simulink model "MatchedfilterImproved"  (R2023b)
settings: Solver=VariableStepAuto  StartTime=0.0  StopTime=4000/fs  RelTol=1e-3
PreLoadFcn:
  | fs = 16e6;
  | 
  | % Test tone
  | f = 0.2*16e6;
  | 
  | % Parameters
  | N = 2048;
  | n = 0:N-1;
  | 
  | % Windows
  | Hamming = 0.54 - 0.46 * cos(2*pi*n/N);
  | Norm_Ham = sum(Hamming);
  | Hanning = 0.5 * (1 + cos(2*pi*n/N));
  | Norm_Han = sum(Hanning);
values from neighbouring files (symbols this model uses):
  template = fliplr(conj(template))    [MF_startup.m]
libraries: hdlBasic x46, hdlDSPIP x3, hdlsllib x2, vmcUtilities x1
settings Model: Creator=qsb20164  LastModifiedBy=jojok
settings DebuggingCC: UnconnectedInputMsg=warning  UnconnectedOutputMsg=warning  UnconnectedLineMsg=warning
settings ModelReferenceCC: EnableRefExpFcnMdlSchedulingChecks=on
settings RTWCC: DLArmComputeVersion=19.05

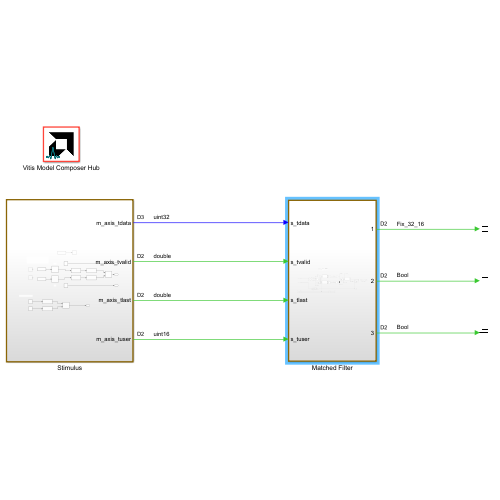
[thumbnail: Simulink's stored preview of the top-level diagram]
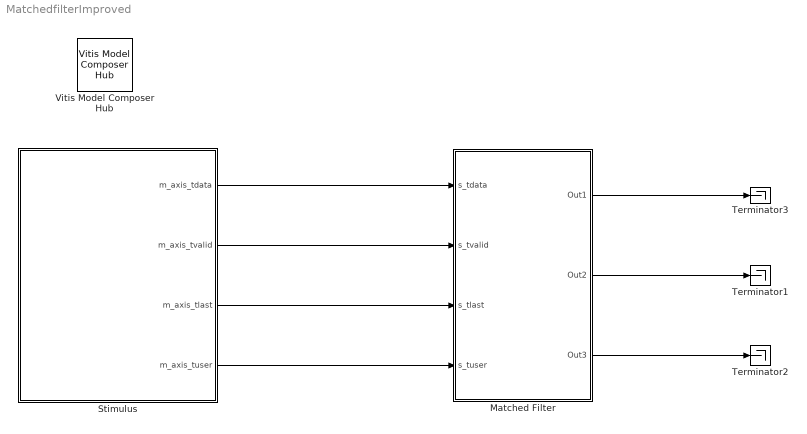
== system MatchedfilterImproved ==
  Matched Filter : Subsystem
  Stimulus : Subsystem
  Terminator1 : Terminator
  Terminator2 : Terminator
  Terminator3 : Terminator
  Vitis Model Composer Hub : vmcUtilities/Vitis Model Composer Hub  Tag=genX  CodeGeneration=off  SubsystemName=Matched Filter  DUTSubsystemName=Matched Filter  CompilationType=HDLCompilation  ExportTypeV2=IP Catalog  TargetDirectory=./ImprovedMFnetlist\ip\Matched_Filter\src  exportDesign=on  analyzeDesign=off  validateDesignOnHw=off  ExportType=HDL  IpVendor=xilinx.com  IpLibrary=hls  IpVersion=1.0  IpHWLanguage=Verilog  AieCompilerOptions={}  AieSimulatorOptions={}  CreateTestbench=off  TestbenchStackSize=10  RunRtlSim=off  RunCSim=off  RunAieSim=off  AieSimTimeout=50000  RunAieSimProfiling=off  LaunchVitisAnalyzer=off  PlotOutput=off  RunX86Sim=off  X86SimTimeout=10  GenHwImage=off  GenLibadfXo=on  GenHwValidationCode=off  PlatformType=Not Specified  HwSystemType=Baremetal  HwValidationTarget=hw  ProjDevice=xczu28dr-ffvg1517-2-e  ProjDevicePart=xczu28dr-ffvg1517-2-e  SamplePeriod=-1  ClockFrequency=200  DataPathParallelism=1  xilinxfamily=zynquplusRFSOC  part=xczu28dr  speed=-2-e  package=ffvg1517  directory=./netlist\ip\Matched_Filter\src  testbench=off  incr_netlist=off  synthesis_tool=Vivado  clock_wrapper=Clock Enables  dbl_ovrd=According to Block Masks  dcm_input_clock_period=10  sysclk_period=4  simulink_period=1/(2*fs)  eval_field=0  IPInfoJsonString="{\"HDLSubsystem\":{\"SubsystemName\":\"Matched_Filter\",\"IPName\":\"Matched_Filter\",\"IPLibrary\":\"VMC\",\"IPVendor\":\"User Company\",\"IPVersion\":\"1.0\",\"TargetDirectory\":\"./ImprovedMFnetlist\",\"SubsystemDir\":\"./ImprovedMFnetlist\\\\ip\\\\Matched_Filter\"},\"SubsystemTag\":\"HDLNode\"}"  LogFileName=''  NThreads=4
  wires:
  Stimulus/1(m_axis_tdata) -> Matched Filter/1(s_tdata)
  Stimulus/2(m_axis_tvalid) -> Matched Filter/2(s_tvalid)
  Stimulus/3(m_axis_tlast) -> Matched Filter/3(s_tlast)
  Matched Filter/1(Out1) -> Terminator3/1
  Matched Filter/2(Out2) -> Terminator1/1
  Matched Filter/3(Out3) -> Terminator2/1
  Stimulus/4(m_axis_tuser) -> Matched Filter/4(s_tuser)

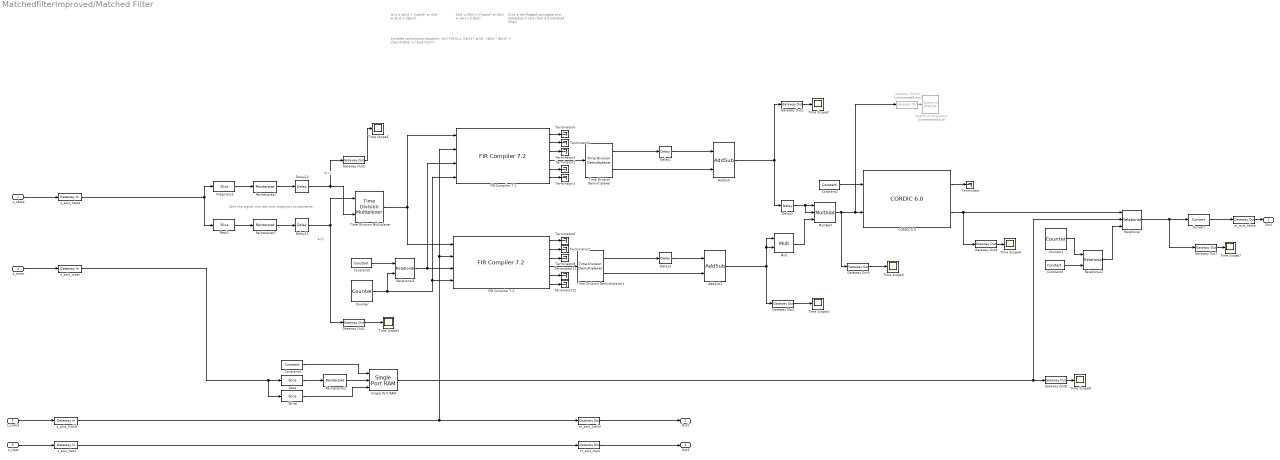
== system MatchedfilterImproved/Matched Filter ==
  note: a[n]
  note: b[n]
  note: h[n] is the flipped conjugate
      | of a template in x[n]
      | (this is a matched filter)
  note: h[n] = hl[n] + j(hq[n])
      | or
      | h[n] = c[n] + j(d[n])
  note: x[n] = xl[n] + j(xq[n])
      | or
      | x[n] = a[n] + j(b[n])
  note: Complex convolution equation:
      |
      | x[n] * h[n] = ((a[n] * c[n]) - (b[n] * d[n])) + j((a[n]*d[n]) + (b[n]*c[n]))
  note: Split the signal into real and imaginary components
  s_tdata : Inport
  s_tvalid : Inport  Port=2
  s_tlast : Inport  Port=3
  s_tuser : Inport  Port=4
  AddSub : hdlBasic/AddSub  mode=Subtraction  use_carryin=off  use_carryout=off  en=off  latency=1  precision=Full  arith_type=Unsigned  n_bits=16  bin_pt=14  quantization=Truncate  overflow=Wrap  use_behavioral_HDL=off  hw_selection=Fabric  pipelined=off  XmcBlockStatus=1  maskContainerNames=tabcontainer1  block_type=addsub  block_config=sysgen:Addsub_config
  AddSub1 : hdlBasic/AddSub  mode=Addition  use_carryin=off  use_carryout=off  en=off  latency=1  precision=Full  arith_type=Unsigned  n_bits=16  bin_pt=14  quantization=Truncate  overflow=Wrap  use_behavioral_HDL=off  hw_selection=Fabric  pipelined=off  XmcBlockStatus=1  maskContainerNames=tabcontainer1  block_type=addsub  block_config=sysgen:Addsub_config
  CORDIC 6.0 : hdlDSPIP/CORDIC 6.0   functional_selection=Square_Root  architectural_configuration=Parallel  pipelining_mode=Maximum  data_format=UnsignedInteger  phase_format=Radians  input_width=46  output_width=24  round_mode=Truncate  iterations=0  precision=0  compensation_scaling=No_Scale_Compensation  coarse_rotation=off  aclken=off  aresetn=off  out_tready=off  cartesian_has_tuser=off  cartesian_has_tlast=off  cartesian_tuser_width=1  phase_has_tuser=off  phase_has_tlast=off  phase_tuser_width=1  out_tlast_behv=Null  flow_control=NonBlocking  optimize_goal=Resources  trim_axipin_name=on  simulation_type=hybrid_sim  simulation_model=sysgen:cordic_v6_0  data_path_portlist={'s_axis_cartesian_tdata_imag', 's_axis_cartesian_tdata_real', 's_axis_phase_tdata_phase', 'm_axis_dout_tdata_imag', 'm_axis_dout_tdata_real', 'm_axis_dout_tdata_phase','m_axis_dout_tdata'}  ip_name=CORDIC  ip_version=6.0  dsptool_ready=true  ipcore_usecache=true  ipcore_useipmodelcache=true  wrapper_available=true  port_translation_map={ 'aclken' => 'en', 'aresetn' => 'rst' }  XmcBlockStatus=1  maskContainerNames=group15  block_type=cordic_v6_0  block_config=sysgen:rodinimport_config  block_width=800
  Constant2 : hdlBasic/Constant  const=1.0  gui_display_data_type=Boolean  arith_type=Boolean  n_bits=16  bin_pt=14  preci_type=Single  exp_width=8  frac_width=24  explicit_period=off  period=1  XmcBlockStatus=1  maskContainerNames=tabcontainer1  block_type=constant  block_config=sysgen:Constant_config
  Constant3 : hdlBasic/Constant  const=6  gui_display_data_type=Fixed-point  arith_type=Unsigned  n_bits=16  bin_pt=0  preci_type=Single  exp_width=8  frac_width=24  explicit_period=off  period=1  XmcBlockStatus=1  maskContainerNames=tabcontainer1  block_type=constant  block_config=sysgen:Constant_config
  Constant4 : hdlBasic/Constant  const=1.0  gui_display_data_type=Fixed-point  arith_type=Unsigned  n_bits=1  bin_pt=0  preci_type=Single  exp_width=8  frac_width=24  explicit_period=off  period=1  XmcBlockStatus=1  maskContainerNames=tabcontainer1  block_type=constant  block_config=sysgen:Constant_config
  Constant5 : hdlBasic/Constant  const=1.0  gui_display_data_type=Fixed-point  arith_type=Signed (2's comp)  n_bits=16  bin_pt=14  preci_type=Single  exp_width=8  frac_width=24  explicit_period=off  period=1  XmcBlockStatus=1  maskContainerNames=tabcontainer1  block_type=constant  block_config=sysgen:Constant_config
  Convert : hdlBasic/Convert  gui_display_data_type=Fixed-point  arith_type=Signed (2's comp)  n_bits=32  bin_pt=16  float_type=Single  exp_bits=8  fraction_bits=24  quantization=Truncate  overflow=Wrap  en=off  latency=1  pipeline=off  XmcBlockStatus=1  maskContainerNames=group2  block_type=convert  block_config=sysgen:Convert_config  block_width=595  block_height=885
  Counter : hdlBasic/Counter  cnt_type=Count limited  cnt_to=1  operation=Up  start_count=0  cnt_by_val=1  arith_type=Unsigned  n_bits=1  bin_pt=0  load_pin=off  rst=off  en=off  explicit_period=Explicit  period=1/fs  use_behavioral_HDL=off  implementation=Fabric  XmcBlockStatus=1  maskContainerNames=group1  block_type=counter  block_config=sysgen:Counter_config  block_width=531  block_height=1023
  Counter1 : hdlBasic/Counter  cnt_type=Count limited  cnt_to=6  operation=Up  start_count=0  cnt_by_val=1  arith_type=Unsigned  n_bits=16  bin_pt=0  load_pin=off  rst=off  en=off  explicit_period=Explicit  period=1/fs  use_behavioral_HDL=off  implementation=Fabric  XmcBlockStatus=1  maskContainerNames=group1  block_type=counter  block_config=sysgen:Counter_config  block_width=531  block_height=1023
  Data : hdlBasic/Slice  nbits=15  boolean_output=off  mode=Upper Bit Location + Width  bit1=15  base1=LSB of Input  bit0=16*8-(16*1)  base0=LSB of Input  XmcBlockStatus=1  maskContainerNames=group1  block_type=slice  block_config=sysgen:Slice_config
  Delay{1,3,11..12} (4 alike) : hdlBasic/Delay  rst=off  en=off  latency=1  reg_retiming=off  XmcBlockStatus=1  maskContainerNames=group1  block_type=delay  block_config=sysgen:Delay_config
  Delay2 : hdlBasic/Delay  rst=off  en=off  latency=3  reg_retiming=off  XmcBlockStatus=1  maskContainerNames=group1  block_type=delay  block_config=sysgen:Delay_config
  FIR Compiler 7.1 : hdlDSPIP/FIR Compiler 7.2   coefficientvector=[real(template), imag(template)]  coefficient_sets=2  coefficient_reload=off  filter_type=Single_Rate  rate_change_type=Integer  interpolation_rate=1  decimation_rate=1  zero_pack_factor=1  channel_sequence=Basic  number_channels=2  pattern_list='P4-0,P4-1,P4-2,P4-3,P4-4'  number_paths=1  ratespecification=Maximum_Possible  sampleperiod=1  hardwareoversamplingrate=1  coefficient_sign=Signed  quantization=Quantize_Only  coefficient_width=16  bestprecision=off  coefficient_fractional_bits=14  coefficient_structure=Inferred  output_rounding_mode=Full_Precision  output_width=36  filter_architecture=Systolic_Multiply_Accumulate  optimization_goal=Area  optimization_list='None'  data_buffer_type=Automatic  coefficient_buffer_type=Automatic  input_buffer_type=Automatic  output_buffer_type=Automatic  preference_for_other_storage=Automatic  multi_column_support=Automatic  columnconfig='84'  inter_column_pipe_length=4  data_has_tlast=Not_Required  m_data_has_tready=off  s_data_has_fifo=off  s_data_has_tuser=Not_Required  m_data_has_tuser=Not_Required  s_config_sync_mode=On_Vector  s_config_method=By_Channel  num_reload_slots=1  has_aclken=off  has_aresetn=off  reset_data_vector=on  trim_axipin_name=on  simulation_type=hybrid_sim  simulation_model=sysgen:xfirv7_2_cmodel  data_path_portlist={ 's_axis_data_tdata', 'm_axis_data_tdata' }  passband_min=0.0  passband_max=0.5  stopband_min=0.5  stopband_max=1.0  filter_selection=1  gui_behaviour='Sysgen_GUI'  data_sign=Signed  data_width=16  data_fractional_bits=0  data_tuser_width=1  wrapper_available=true  ip_wrap_arbitrary_binary_point=true  ip_name=FIR Compiler  ip_version=7.2  dsptool_ready=true  ipcore_usecache=true  ipcore_useipmodelcache=true  port_translation_map={ 'aclken' => 'en', 'aresetn' => 'rst' }  run_core_at_system_period=true  ipcore_xco_need_fpga_part=true  ipcore_fpga_part=[]  XmcBlockStatus=1  maskContainerNames=tabcontainer1  block_type=fir_compiler_v7_2  block_config=sysgen:rodinimport_config  block_width=820  block_height=600
  FIR Compiler 7.2 : hdlDSPIP/FIR Compiler 7.2   coefficientvector=[imag(template), real(template)]  coefficient_sets=2  coefficient_reload=off  filter_type=Single_Rate  rate_change_type=Integer  interpolation_rate=1  decimation_rate=1  zero_pack_factor=1  channel_sequence=Basic  number_channels=2  pattern_list='P4-0,P4-1,P4-2,P4-3,P4-4'  number_paths=1  ratespecification=Maximum_Possible  sampleperiod=1  hardwareoversamplingrate=1  coefficient_sign=Signed  quantization=Quantize_Only  coefficient_width=16  bestprecision=off  coefficient_fractional_bits=14  coefficient_structure=Inferred  output_rounding_mode=Full_Precision  output_width=36  filter_architecture=Systolic_Multiply_Accumulate  optimization_goal=Area  optimization_list='None'  data_buffer_type=Automatic  coefficient_buffer_type=Automatic  input_buffer_type=Automatic  output_buffer_type=Automatic  preference_for_other_storage=Automatic  multi_column_support=Automatic  columnconfig='84'  inter_column_pipe_length=4  data_has_tlast=Not_Required  m_data_has_tready=off  s_data_has_fifo=off  s_data_has_tuser=Not_Required  m_data_has_tuser=Not_Required  s_config_sync_mode=On_Vector  s_config_method=By_Channel  num_reload_slots=1  has_aclken=off  has_aresetn=off  reset_data_vector=on  trim_axipin_name=on  simulation_type=hybrid_sim  simulation_model=sysgen:xfirv7_2_cmodel  data_path_portlist={ 's_axis_data_tdata', 'm_axis_data_tdata' }  passband_min=0.0  passband_max=0.5  stopband_min=0.5  stopband_max=1.0  filter_selection=1  gui_behaviour='Sysgen_GUI'  data_sign=Signed  data_width=16  data_fractional_bits=0  data_tuser_width=1  wrapper_available=true  ip_wrap_arbitrary_binary_point=true  ip_name=FIR Compiler  ip_version=7.2  dsptool_ready=true  ipcore_usecache=true  ipcore_useipmodelcache=true  port_translation_map={ 'aclken' => 'en', 'aresetn' => 'rst' }  run_core_at_system_period=true  ipcore_xco_need_fpga_part=true  ipcore_fpga_part=[]  XmcBlockStatus=1  maskContainerNames=tabcontainer1  block_type=fir_compiler_v7_2  block_config=sysgen:rodinimport_config  block_width=820  block_height=600
  Gateway Out{1..8} (8 alike) : hdlBasic/Gateway Out  inherit_from_input=off  hdl_port=off  rows=1  columns=1  UseAsDAC=off  DACChannel='1'  interface=None  automatic_assignment=on  address_offset=hex2dec('00')  intf_name=''  intf_description=''  timing_constraint=None  locs_specified=off  LOCs={}  io_standard={}  XmcBlockStatus=1  maskContainerNames=group4  block_type=gatewayout  block_config=sysgen:gateway_out_config  block_width_w=590  block_height_w=620  block_width=620  block_height=750
  Gateway Out10 : hdlBasic/Gateway Out  Commented=on  inherit_from_input=off  hdl_port=off  rows=1  columns=1  UseAsDAC=off  DACChannel='1'  interface=None  automatic_assignment=on  address_offset=hex2dec('00')  intf_name=''  intf_description=''  timing_constraint=None  locs_specified=off  LOCs={}  io_standard={}  XmcBlockStatus=1  maskContainerNames=group4  block_type=gatewayout  block_config=sysgen:gateway_out_config  block_width_w=590  block_height_w=620  block_width=620  block_height=750
  Imaginary1 : hdlBasic/Slice  nbits=16  boolean_output=off  mode=Two Bit Locations  bit1=31  base1=LSB of Input  bit0=16  base0=LSB of Input  XmcBlockStatus=1  maskContainerNames=group1  block_type=slice  block_config=sysgen:Slice_config
  Mult : hdlBasic/Mult  precision=Full  arith_type="Signed  (2's comp)"  n_bits=16  bin_pt=14  quantization=Truncate  overflow=Wrap  en=off  latency=3  use_behavioral_HDL=off  opt=Speed  use_embedded=on  optimum_pipeline=off  pipeline=on  use_rpm=on  placement_style=Triangular  XmcBlockStatus=1  maskContainerNames=group1  block_type=mult  block_config=sysgen:Mult_config  block_width=598  block_height=876
  MultAdd : hdlBasic/MultAdd  mode=Addition  en=off  latency=0  precision=User Defined  arith_type=Unsigned  n_bits=48  bin_pt=0  XmcBlockStatus=1  maskContainerNames=tabcontainer1  block_type=multadd  block_config=sysgen:MultAdd_config
  Real1 : hdlBasic/Slice  nbits=16  boolean_output=off  mode=Two Bit Locations  bit1=15  base1=LSB of Input  bit0=0  base0=LSB of Input  XmcBlockStatus=1  maskContainerNames=group1  block_type=slice  block_config=sysgen:Slice_config
  Reinterpret1 : hdlBasic/Reinterpret  force_arith_type=on  arith_type="Signed  (2's comp)"  force_bin_pt=on  bin_pt=15  XmcBlockStatus=1  maskContainerNames=group1  block_type=reinterpret  block_config=sysgen:Reinterpret_config
  Reinterpret2 : hdlBasic/Reinterpret  force_arith_type=on  arith_type=Unsigned  force_bin_pt=on  bin_pt=6  XmcBlockStatus=1  maskContainerNames=group1  block_type=reinterpret  block_config=sysgen:Reinterpret_config
  Reinterpret7 : hdlBasic/Reinterpret  force_arith_type=on  arith_type="Signed  (2's comp)"  force_bin_pt=on  bin_pt=15  XmcBlockStatus=1  maskContainerNames=group1  block_type=reinterpret  block_config=sysgen:Reinterpret_config
  Relational : hdlBasic/Relational  mode=a>b  op_type=Bool  en=on  latency=1  XmcBlockStatus=1  maskContainerNames=tabcontainer1  block_type=relational  block_config=sysgen:Relational_config
  Relational1 : hdlBasic/Relational  mode=a=b  op_type=Bool  en=off  latency=1  XmcBlockStatus=1  maskContainerNames=tabcontainer1  block_type=relational  block_config=sysgen:Relational_config
  Relational2 : hdlBasic/Relational  mode=a=b  op_type=Bool  en=off  latency=1  XmcBlockStatus=1  maskContainerNames=tabcontainer1  block_type=relational  block_config=sysgen:Relational_config
  Single Port RAM : hdlBasic/Single Port RAM  depth=2  initVector=[0 0]  distributed_mem=Distributed memory  write_mode=Read After Write  rst=off  init_reg=0  en=off  optimize_latency=on  latency=1  optimize=Area  dbl_ovrd=off  simulation_type=fast_sim  XmcBlockStatus=1  maskContainerNames=tabcontainer1  block_type=spram  block_config=sysgen:SPRAM_config
  Spectrum Analyzer1 : SpectrumAnalyzer  Commented=on  SampleRate=16000000  AxesScaling=Manual  Span=16000000  StartFrequency=-8000000  StopFrequency=8000000  AveragingMethod=Exponential  YLimits=[-85.389381881293900278,31.375193648210043307]  DefaultConfigurationName=spbscopes.SpectrumAnalyzerBlockCfg  IsFrequencyInputMode=0  FrequencyVectorPort=0  FrequencyVectorFromPort=0  FrequencyInputRBWPort=0  FrequencyInputRBWFromPort=0
  Terminator{,1..8,11..12} (11 alike) : Terminator
  Time Scope{1..8} (8 alike) : Scope
  Time Division Demultiplexer : hdlBasic/Time Division Demultiplexer  frame_pattern=[1 1]  impl_style=Multiple Channel  vin=off  explicit_period=off  period=1  XmcBlockStatus=1  maskContainerNames=group2  block_type=tdd  block_config=sysgen:TDD_config
  Time Division Demultiplexer1 : hdlBasic/Time Division Demultiplexer  frame_pattern=[1 1]  impl_style=Multiple Channel  vin=off  explicit_period=off  period=1  XmcBlockStatus=1  maskContainerNames=group2  block_type=tdd  block_config=sysgen:TDD_config
  Time Division Multiplexer : hdlBasic/Time Division Multiplexer  inputs=2  vin=off  Optimization=Resource  explicit_period=off  period=1  XmcBlockStatus=1  maskContainerNames=group3  block_type=tdm  block_config=sysgen:TDM_config
  Write : hdlBasic/Slice  nbits=1  boolean_output=on  mode=Upper Bit Location + Width  bit1=0  base1=LSB of Input  bit0=16*8-(16*1)  base0=LSB of Input  XmcBlockStatus=1  maskContainerNames=group1  block_type=slice  block_config=sysgen:Slice_config
  m_axis_tdata : hdlBasic/Gateway Out  inherit_from_input=on  hdl_port=on  rows=1  columns=1  UseAsDAC=off  DACChannel='1'  interface=None  automatic_assignment=on  address_offset=hex2dec('00')  intf_name=''  intf_description=''  timing_constraint=None  locs_specified=off  LOCs={}  io_standard={}  XmcBlockStatus=1  maskContainerNames=group4  block_type=gatewayout  block_config=sysgen:gateway_out_config  block_width_w=590  block_height_w=620  block_width=620  block_height=750
  m_axis_tlast : hdlBasic/Gateway Out  inherit_from_input=on  hdl_port=on  rows=1  columns=1  UseAsDAC=off  DACChannel='1'  interface=None  automatic_assignment=on  address_offset=hex2dec('00')  intf_name=''  intf_description=''  timing_constraint=None  locs_specified=off  LOCs={}  io_standard={}  XmcBlockStatus=1  maskContainerNames=group4  block_type=gatewayout  block_config=sysgen:gateway_out_config  block_width_w=590  block_height_w=620  block_width=620  block_height=750
  m_axis_tvalid : hdlBasic/Gateway Out  inherit_from_input=on  hdl_port=on  rows=1  columns=1  UseAsDAC=off  DACChannel='1'  interface=None  automatic_assignment=on  address_offset=hex2dec('00')  intf_name=''  intf_description=''  timing_constraint=None  locs_specified=off  LOCs={}  io_standard={}  XmcBlockStatus=1  maskContainerNames=group4  block_type=gatewayout  block_config=sysgen:gateway_out_config  block_width_w=590  block_height_w=620  block_width=620  block_height=750
  s_axis_tdata : hdlBasic/Gateway In  gui_display_data_type=Fixed-point  arith_type=Unsigned  n_bits=32  bin_pt=0  preci_type=Single  exp_width=8  frac_width=24  rows=1  columns=1  quantization="Round  (unbiased: +/- Inf)"  overflow=Saturate  period=1/fs  UseAsADC=off  ADCChannel='1'  interface=None  automatic_assignment=on  address_offset=hex2dec('00')  intf_name=''  intf_description=''  default_value=0  timing_constraint=None  locs_specified=off  LOCs={}  io_standard={}  inherit_from_input=off  hdl_port=on  XmcBlockStatus=1  maskContainerNames=group4  block_type=gatewayin  block_config=sysgen:gateway_in_config  block_width_w=590  block_height_w=620  block_width=640  block_height=850
  s_axis_tlast : hdlBasic/Gateway In  gui_display_data_type=Boolean  arith_type=Boolean  n_bits=16  bin_pt=14  preci_type=Single  exp_width=8  frac_width=24  rows=1  columns=1  quantization="Round  (unbiased: +/- Inf)"  overflow=Saturate  period=1/fs  UseAsADC=off  ADCChannel='1'  interface=None  automatic_assignment=on  address_offset=hex2dec('00')  intf_name=''  intf_description=''  default_value=0  timing_constraint=None  locs_specified=off  LOCs={}  io_standard={}  inherit_from_input=off  hdl_port=on  XmcBlockStatus=1  maskContainerNames=group4  block_type=gatewayin  block_config=sysgen:gateway_in_config  block_width_w=590  block_height_w=620  block_width=640  block_height=850
  s_axis_tuser : hdlBasic/Gateway In  gui_display_data_type=Fixed-point  arith_type=Unsigned  n_bits=16  bin_pt=0  preci_type=Single  exp_width=8  frac_width=24  rows=1  columns=1  quantization="Round  (unbiased: +/- Inf)"  overflow=Saturate  period=1/fs  UseAsADC=off  ADCChannel='1'  interface=None  automatic_assignment=on  address_offset=hex2dec('00')  intf_name=''  intf_description=''  default_value=0  timing_constraint=None  locs_specified=off  LOCs={}  io_standard={}  inherit_from_input=off  hdl_port=on  XmcBlockStatus=1  maskContainerNames=group4  block_type=gatewayin  block_config=sysgen:gateway_in_config  block_width_w=590  block_height_w=620  block_width=640  block_height=850
  s_axis_tvalid : hdlBasic/Gateway In  gui_display_data_type=Boolean  arith_type=Boolean  n_bits=16  bin_pt=14  preci_type=Single  exp_width=8  frac_width=24  rows=1  columns=1  quantization="Round  (unbiased: +/- Inf)"  overflow=Saturate  period=1/fs  UseAsADC=off  ADCChannel='1'  interface=None  automatic_assignment=on  address_offset=hex2dec('00')  intf_name=''  intf_description=''  default_value=0  timing_constraint=None  locs_specified=off  LOCs={}  io_standard={}  inherit_from_input=off  hdl_port=on  XmcBlockStatus=1  maskContainerNames=group4  block_type=gatewayin  block_config=sysgen:gateway_in_config  block_width_w=590  block_height_w=620  block_width=640  block_height=850
  Out1 : Outport
  Out2 : Outport  Port=2
  Out3 : Outport  Port=3
  wires:
  m_axis_tvalid/1 -> Out2/1
  s_tlast/1 -> s_axis_tlast/1
  s_axis_tvalid/1 -> FIR Compiler 7.1/2, FIR Compiler 7.2/2, m_axis_tvalid/1
  s_axis_tlast/1 -> m_axis_tlast/1
  m_axis_tdata/1 -> Out1/1
  s_tvalid/1 -> s_axis_tvalid/1
  s_tdata/1 -> s_axis_tdata/1
  m_axis_tlast/1 -> Out3/1
  Imaginary1/1 -> Reinterpret1/1
  Real1/1 -> Reinterpret7/1
  Reinterpret1/1 -> Delay12/1
  Reinterpret7/1 -> Delay11/1
  Delay12/1 -> Gateway Out5/1, Time Division Multiplexer/2
  AddSub1/1 -> Mult/2, Mult/1, Gateway Out3/1
  Delay11/1 -> Time Division Multiplexer/1, Gateway Out1/1
  AddSub/1 -> Delay2/1, Gateway Out2/1
  Gateway Out1/1 -> Time Scope1/1
  Gateway Out2/1 -> Time Scope2/1
  Gateway Out3/1 -> Time Scope3/1
  CORDIC 6.0/2 -> Relational/1, Gateway Out4/1
  Gateway Out4/1 -> Time Scope4/1
  Gateway Out5/1 -> Time Scope5/1
  Mult/1 -> MultAdd/3
  MultAdd/1 -> Gateway Out10/1, CORDIC 6.0/2, Gateway Out6/1
  Constant2/1 -> CORDIC 6.0/1
  CORDIC 6.0/1 -> Terminator/1
  Gateway Out6/1 -> Time Scope6/1
  Relational/1 -> Convert/1, Gateway Out7/1
  Gateway Out7/1 -> Time Scope7/1
  Constant4/1 -> Single Port RAM/1
  Reinterpret2/1 -> Single Port RAM/2
  Data/1 -> Reinterpret2/1
  Write/1 -> Single Port RAM/3
  s_axis_tuser/1 -> Data/1, Write/1
  s_tuser/1 -> s_axis_tuser/1
  Gateway Out8/1 -> Time Scope8/1
  Single Port RAM/1 -> Relational/2, Gateway Out8/1
  Counter1/1 -> Relational2/1
  Constant3/1 -> Relational2/2
  Relational2/1 -> Relational/3
  s_axis_tdata/1 -> Real1/1, Imaginary1/1
  Gateway Out10/1 -> Spectrum Analyzer1/1
  Time Division Multiplexer/1 -> FIR Compiler 7.2/1, FIR Compiler 7.1/1
  Counter/1 -> FIR Compiler 7.2/4, FIR Compiler 7.1/4, Relational1/2
  Constant5/1 -> Relational1/1
  Relational1/1 -> FIR Compiler 7.2/3, FIR Compiler 7.1/3
  FIR Compiler 7.1/4 -> Time Division Demultiplexer/1
  FIR Compiler 7.1/6 -> Terminator1/1
  FIR Compiler 7.2/4 -> Time Division Demultiplexer1/1
  FIR Compiler 7.1/5 -> Terminator2/1
  FIR Compiler 7.1/3 -> Terminator3/1
  FIR Compiler 7.1/2 -> Terminator4/1
  FIR Compiler 7.1/1 -> Terminator5/1
  FIR Compiler 7.2/1 -> Terminator6/1
  FIR Compiler 7.2/2 -> Terminator7/1
  FIR Compiler 7.2/3 -> Terminator8/1
  FIR Compiler 7.2/5 -> Terminator11/1
  FIR Compiler 7.2/6 -> Terminator12/1
  Delay2/1 -> MultAdd/2, MultAdd/1
  Convert/1 -> m_axis_tdata/1
  Time Division Demultiplexer/1 -> Delay1/1
  Time Division Demultiplexer1/1 -> Delay3/1
  Time Division Demultiplexer/2 -> AddSub/2
  Time Division Demultiplexer1/2 -> AddSub1/2
  Delay1/1 -> AddSub/1
  Delay3/1 -> AddSub1/1

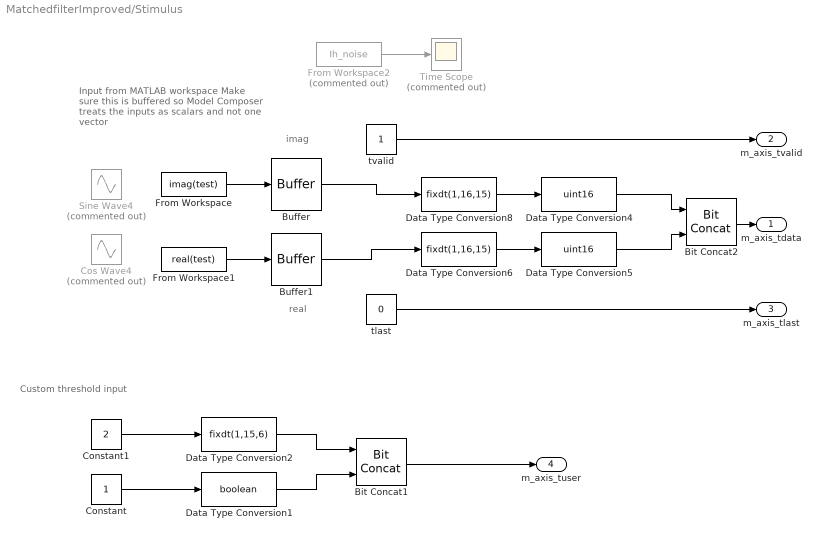
== system MatchedfilterImproved/Stimulus ==
  note: Input from MATLAB workspace
      | Make sure this is buffered so Model
      | Composer treats the inputs as scalars
      | and not one vector
  note: Custom threshold input
  note: real
  note: imag
  Bit Concat1 : hdlsllib/Logic and Bit Operations/Bit Concat  numInputs=2
  Bit Concat2 : hdlsllib/Logic and Bit Operations/Bit Concat  numInputs=2
  Buffer : Buffer  N=1  OutputFrames=off
  Buffer1 : Buffer  N=1  OutputFrames=off
  Constant : Constant  SampleTime=1/fs
  Constant1 : Constant  Value=2  SampleTime=1/fs
  Cos Wave4 : Sin  Commented=on  Amplitude=0.4  Frequency=f*pi  Phase=pi/2  SampleTime=1/fs
  Data Type Conversion1 : DataTypeConversion  OutDataTypeStr=boolean  RndMeth=Floor
  Data Type Conversion2 : DataTypeConversion  OutDataTypeStr=fixdt(1,15,6)  RndMeth=Floor
  Data Type Conversion4 : DataTypeConversion  OutDataTypeStr=uint16  ConvertRealWorld=Stored Integer (SI)  SaturateOnIntegerOverflow=off  RndMeth=Floor
  Data Type Conversion5 : DataTypeConversion  OutDataTypeStr=uint16  ConvertRealWorld=Stored Integer (SI)  SaturateOnIntegerOverflow=off  RndMeth=Floor
  Data Type Conversion6 : DataTypeConversion  OutDataTypeStr=fixdt(1,16,15)  RndMeth=Floor
  Data Type Conversion8 : DataTypeConversion  OutDataTypeStr=fixdt(1,16,15)  RndMeth=Floor
  From Workspace : FromWorkspace  VariableName=imag(test)  OutDataTypeStr=double  SampleTime=1500/fs
  From Workspace1 : FromWorkspace  VariableName=real(test)  OutDataTypeStr=double  SampleTime=1500/fs
  From Workspace2 : FromWorkspace  Commented=on  VariableName=Ih_noise  SampleTime=1500/fs  OutputAfterFinalValue=Setting to zero
  Sine Wave4 : Sin  Commented=on  Amplitude=0.4  Frequency=f*pi  SampleTime=1/fs
  Time Scope : Scope  Commented=on
  tlast : Constant  Value=0  SampleTime=1/fs
  tvalid : Constant  SampleTime=1/fs
  m_axis_tdata : Outport
  m_axis_tvalid : Outport  Port=2
  m_axis_tlast : Outport  Port=3
  m_axis_tuser : Outport  Port=4
  wires:
  Data Type Conversion6/1 -> Data Type Conversion5/1
  Data Type Conversion4/1 -> Bit Concat2/1
  Data Type Conversion8/1 -> Data Type Conversion4/1
  Data Type Conversion5/1 -> Bit Concat2/2
  Bit Concat2/1 -> m_axis_tdata/1
  tvalid/1 -> m_axis_tvalid/1
  tlast/1 -> m_axis_tlast/1
  From Workspace2/1 -> Time Scope/1
  From Workspace/1 -> Buffer/1
  Buffer/1 -> Data Type Conversion8/1
  Buffer1/1 -> Data Type Conversion6/1
  From Workspace1/1 -> Buffer1/1
  Data Type Conversion2/1 -> Bit Concat1/1
  Constant1/1 -> Data Type Conversion2/1
  Constant/1 -> Data Type Conversion1/1
  Data Type Conversion1/1 -> Bit Concat1/2
  Bit Concat1/1 -> m_axis_tuser/1
